simulink subsystem "ADC_DelSig"  (R2025b)
settings: Solver=VariableStepAuto  StartTime=0.0  StopTime=10.0  RelTol=1e-3
undefined symbols (not defined in the file): Decimation_ADC, Ts_ADC, Vref
libraries: dspmlti4 x1
settings Model: Creator=elias  LastModifiedBy=elias

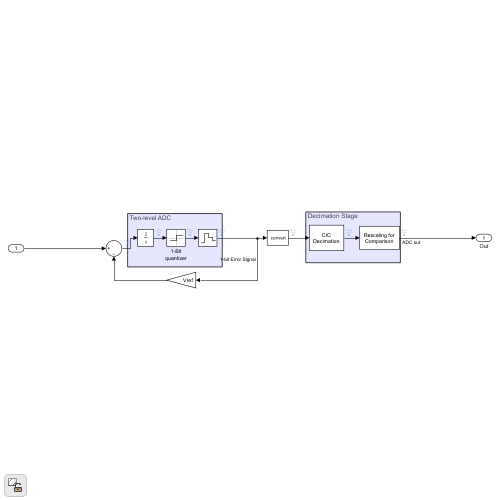
[thumbnail: Simulink's stored preview of the top-level diagram]
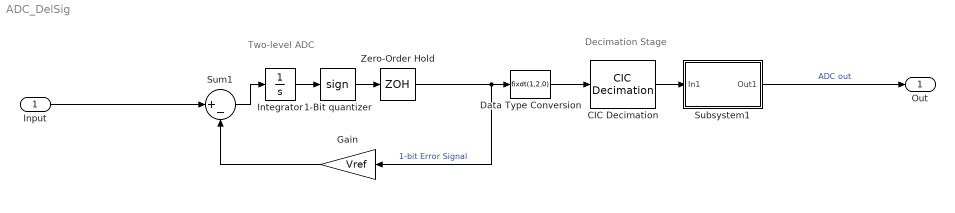
== system ADC_DelSig ==
  note: Decimation Stage
  note: Two-level ADC
  Input : Inport
  1-Bit quantizer : Signum
  CIC Decimation : dspmlti4/CIC Decimation  filtFrom=Dialog parameters  filtobj=Hm_decim  ftype=Decimator  R=Decimation_ADC  M=1  N=5  filterInternals=Full precision  BPS=[32 30 24 20 16 16 16 16 16 16]  FLPS=0  outputWordLength=16  outputFracLength=0  launchFVT=off  framing=Maintain input frame rate  RateOptions=Allow multirate processing
  Data Type Conversion : DataTypeConversion  OutDataTypeStr=fixdt(1,2,0)  SaturateOnIntegerOverflow=off  RndMeth=Floor
  Gain : Gain  Gain=Vref
  Integrator : Integrator
  Subsystem1 : Subsystem
      mask Display: disp('Rescaling for\nComparison')
  Sum1 : Sum  Inputs=|+-  InputSameDT=on  SaturateOnIntegerOverflow=on  OutDataTypeStr=Inherit: Same as first input
  Zero-Order Hold : ZeroOrderHold  SampleTime=Ts_ADC
  Out : Outport
  wires:
  1-Bit quantizer/1 -> Zero-Order Hold/1
  Sum1/1 -> Integrator/1
  Subsystem1/1(Out1) -> Out/1  "ADC out"
  Data Type Conversion/1 -> CIC Decimation/1
  Input/1 -> Sum1/1
  Zero-Order Hold/1 -> Data Type Conversion/1, Gain/1  "1-bit Error Signal"
  Gain/1 -> Sum1/2
  CIC Decimation/1 -> Subsystem1/1(In1)
  Integrator/1 -> 1-Bit quantizer/1

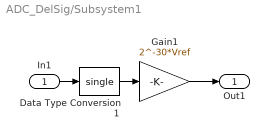
== system ADC_DelSig/Subsystem1 ==
  In1 : Inport
  Data Type Conversion1 : DataTypeConversion  OutDataTypeStr=single  SaturateOnIntegerOverflow=off  RndMeth=Floor
  Gain1 : Gain  Gain=2^-30*Vref  SaturateOnIntegerOverflow=on  OutDataTypeStr=Inherit: Same as input  ParamDataTypeStr=Inherit: Same as input
  Out1 : Outport  VectorParamsAs1DForOutWhenUnconnected=off
  wires:
  Gain1/1 -> Out1/1
  In1/1 -> Data Type Conversion1/1
  Data Type Conversion1/1 -> Gain1/1
